simulink model "d"  (R2024a)
settings: Solver=VariableStepAuto  StartTime=0.0  StopTime=10.0  RelTol=1e-3
settings Model: Creator=ishwo  LastModifiedBy=ishwo

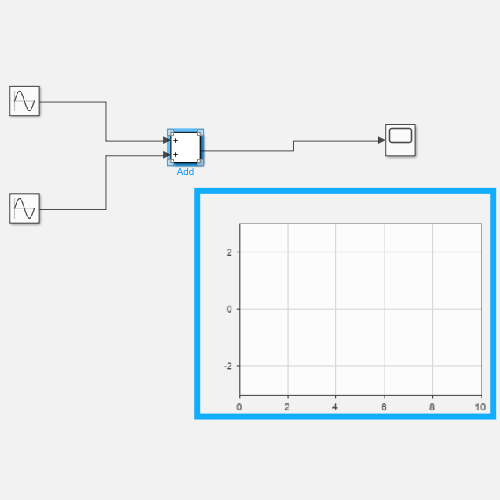
[thumbnail: Simulink's stored preview of the top-level diagram]
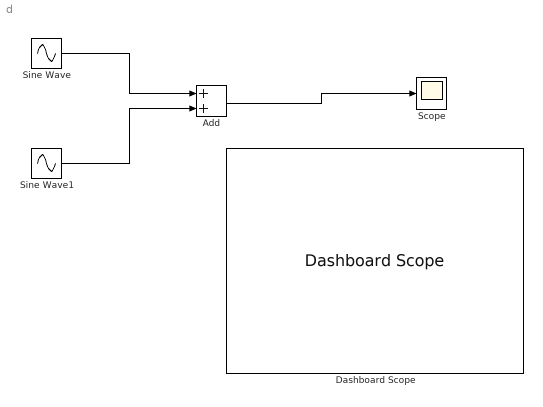
== system d ==
  Add : Sum
  Dashboard Scope : DashboardScope
  Scope : Scope
  Sine Wave : Sin  SampleTime=0
  Sine Wave1 : Sin  SampleTime=0
  wires:
  Sine Wave1/1 -> Add/2
  Sine Wave/1 -> Add/1
  Add/1 -> Scope/1
